simulink model "MicrogridControl"  (R2025b)
settings: Solver=VariableStepAuto  StartTime=0.0  StopTime=8  FixedStep=Ts  RelTol=1e-3
PreLoadFcn:
  | NormalOperation;
  | MicrogridControlParam;
undefined symbols (not defined in the file): base, bessModeInitial, bessSystem, bessVoltage, breakerStatus, DiscIntNeverNeededParam, ee_sli_rtmsupport, event, gcbh, generator, gflInverter, gfmInverter, Inertia, lineInductance, lineResistance, machine, plannedIsland, pmsm, powerLimit, powerQuality, PV, PVInverter, ref, resync, solar, solarInsolationChange, systemFrequency, Ts, windController, windSystem, windTurbine
libraries: nesl_utility x234, ee_lib x174, fl_lib x143, eeGeneralControl x137, simulink x78, eeTransforms x47, slpidlib x23, nesl_utility_internal x12, eePwmGenerator x9, eeSinusoidalMeasurementV2 x9, custom_lib x7, batteryecm_lib x6
(part 1 of 25)
settings Model: SimulationMode=accelerator  Creator=skota  LastModifiedBy=skota
settings DataIOCC: SaveOutput=off  DSMLogging=off  SaveTime=off  ReturnWorkspaceOutputs=off
settings DebuggingCC: MinStepSizeMsg=none  FrameProcessingCompatibilityMsg=none
settings SimscapeCC: SimscapeNormalizeSystem=off

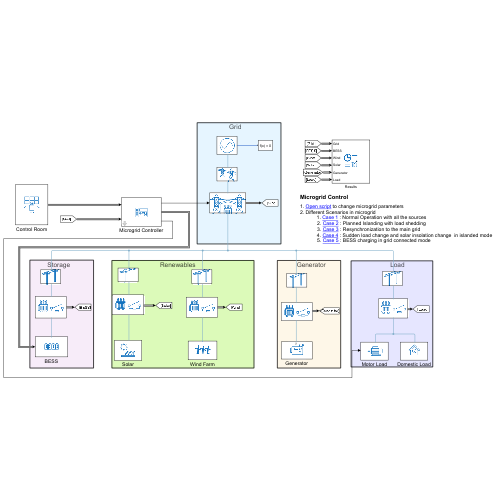
[thumbnail: Simulink's stored preview of the top-level diagram]
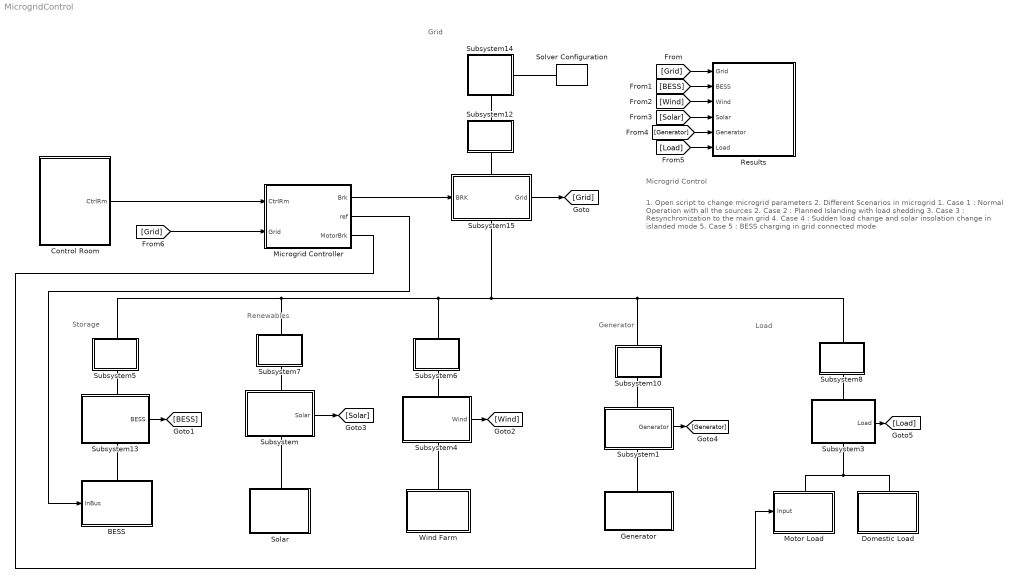
== system MicrogridControl ==
  note: Renewables
  note: Storage
  note: Generator
  note: Load
  note: Grid
  note: 1. Open script to change microgrid parameters
      | 2. Different Scenarios in microgrid
      | 1. Case 1 : Normal Operation with all the sources
      | 2. Case 2 : Planned Islanding with load shedding
      | 3. Case 3 : Resynchronization to the main grid
      | 4. Case 4 : Sudden load change and solar insolation change in islanded mode
      | 5. Case 5 : BESS charging in grid connected mode
  note: Microgrid Control
  BESS : Subsystem
      settings: PortSchema="{\"entries\":[{\"content\":{\"sides\":[{\"content\":{\"connectorIds\":[\"In1\"]},\"type\":\"ConnectorPlacement.EquallySpacedRectSide\",\"uuid\":\"138c02f1-8438-4b9e-be08-ceaf3940f6c7\"},{\"content\":{\"side\":\"RIGHT\"},\"type\":\"ConnectorPlacement.EquallySpacedRectSide\",\"uuid\":\"34af79ec-6d74-4c96-bf33-cc8e5a370ddd\"},{\"content\":{\"connectorIds\":[\"LConn1\"],\"side\":\"TOP\"},\"type\":\"ConnectorPlacement.EquallySpacedRectSide\",\"uuid\":\"48313b6e-1835-49d8-b154-057b5fb517b0\"}]},\"type\":\"ConnectorPlacement.EquallySpacedConnector\",\"uuid\":\"b091f0a3-fffe-4dfb-8622-14774ce4c9e9\"}],\"packageUris\":[\"http://schema.mathworks.com/mf0/Connector/R2020b\"],\"version\":\"1.0\"}"
  Control Room : Subsystem
  Domestic Load : Subsystem
      settings: PortSchema="{\"entries\":[{\"content\":{\"sides\":[{\"content\":{},\"type\":\"ConnectorPlacement.EquallySpacedRectSide\",\"uuid\":\"f8fc4132-7548-4a0f-8659-b0fbdf7b43f6\"},{\"content\":{\"side\":\"RIGHT\"},\"type\":\"ConnectorPlacement.EquallySpacedRectSide\",\"uuid\":\"c12bc99a-3747-4ef2-b83e-90fecef76ea5\"},{\"content\":{\"connectorIds\":[\"LConn1\"],\"side\":\"TOP\"},\"type\":\"ConnectorPlacement.EquallySpacedRectSide\",\"uuid\":\"28127f01-067a-40fd-84ae-a789b4333a80\"}]},\"type\":\"ConnectorPlacement.EquallySpacedConnector\",\"uuid\":\"c6f5d860-c088-4c19-8c9a-849451abfa64\"}],\"packageUris\":[\"http://schema.mathworks.com/mf0/Connector/R2020b\"],\"version\":\"1.0\"}"
  Generator : Subsystem
      settings: PortSchema="{\"entries\":[{\"content\":{\"sides\":[{\"content\":{},\"type\":\"ConnectorPlacement.EquallySpacedRectSide\",\"uuid\":\"0e4bb094-5f01-4715-b678-e6b326bbface\"},{\"content\":{\"side\":\"RIGHT\"},\"type\":\"ConnectorPlacement.EquallySpacedRectSide\",\"uuid\":\"0cb60177-20db-48f9-a9cc-070daf12251a\"},{\"content\":{\"connectorIds\":[\"LConn1\"],\"side\":\"TOP\"},\"type\":\"ConnectorPlacement.EquallySpacedRectSide\",\"uuid\":\"205cef4a-01a9-469e-ade5-58cd4fb704d4\"},{\"content\":{\"side\":\"BOTTOM\"},\"type\":\"ConnectorPlacement.EquallySpacedRectSide\",\"uuid\":\"006e0ade-b558-4494-a2f0-eb5d5c15551c\"}]},\"type\":\"ConnectorPlacement.EquallySpacedConnector\",\"uuid\":\"9a4799c2-8742-4ae9-b78d-c2acced826f3\"}],\"packageUris\":[\"http://schema.mathworks.com/mf0/Connector/R2020b\"],\"version\":\"1.0\"}"
  Microgrid Controller : Subsystem  mask{resynchronization=on, plannedIslanding=on, blackStart=on, kpPLL=40, kiPLL=1000, frequencyPLL=systemFrequency, sampleTimePLL=Ts, pUpperLimit=powerLimit.upper, pLowerLimit=powerLimit.lower, qUpperLimit=powerLimit.upper, qLowerLimit=powerLimit.lower, gridFrequency=systemFrequency, resyncDelay=resync.delay, kpVoltage=resync.kpVoltage, kiVoltage=resync.kiVoltage, voltageThreshold=resync.vThreshold, voltageDroop=resync.vDroop, kpFrequency=resync.kpFrequency, kiFrequency=resync.kiFrequency, frequencyThreshold=resync.fThreshold, kpAngle=resync.kpAngle, kiAngle=resync.kiAngle, angleThreshold=resync.aThreshold, plannedIslandingDelay=plannedIsland.delay, kpActive=plannedIsland.kPActive, kiActive=plannedIsland.kIActive, activeThreshold=plannedIsland.pThreshold, kpReactive=plannedIsland.kPReactive, kiReactive=plannedIsland.kiReactive, reactiveThreshold=plannedIsland.qThreshold, blackStartTime=1000, blackStartFrequency=50, level1=0.1, level2=0.2, level3=0.7, delay1=1, delay2=2, delay3=3, upperVoltagelimit=powerQuality.maxVoltage, lowerVoltageLimit=powerQuality.minVoltage, upperFrequencyLimit=powerQuality.maxFrequency, lowerFrequencyLimit=powerQuality.minFrequency}
      mask prompts: plannedIslanding "Planned Islanding"; blackStart "Black Start"; kpPLL "Proportional Gain"; kiPLL "Integral Gain"; frequencyPLL "Grid Frequency in Hz"; sampleTimePLL "Sample Time in sec"; pUpperLimit "Upper Limit in pu"; pLowerLimit "Lower Limit in pu"; qUpperLimit "Upper Limit in pu"; qLowerLimit "Lower Limit in pu"; gridFrequency "Grid Frequency in Hz"; resyncDelay "Resynchronization delay in sec"; kpVoltage "Proportional Gain"; kiVoltage "Voltage Integral Gain"; voltageThreshold "Threshold"; voltageDroop "Reactive Power Droop"; kpFrequency "Proportional Gain"; kiFrequency "Integral Gain"; frequencyThreshold "Threshold"; kpAngle "Proportional Gain"; kiAngle "Integral Gain"; angleThreshold "Threshold"; plannedIslandingDelay "Delay in sec"; kpActive "Proportional Gain"; kiActive "Integral Gain"; activeThreshold "Threshold"; kpReactive "Proportional Gain"; kiReactive "Integral Gain"; reactiveThreshold "Threshold"; blackStartTime "Black Start Time in sec"; blackStartFrequency "Reference Frequency in Hz"; level1 "Level 1 in pu"; level2 "Level 2 in pu"; level3 "Level 3 in pu"; delay1 "Delay 1 in sec"; delay2 "Delay2 in sec"; delay3 "Delay3 in sec"; upperVoltagelimit "Maximum Voltage in pu"; lowerVoltageLimit "Minimum Voltage in pu"; upperFrequencyLimit "Maximum frequency in Hz"; lowerFrequencyLimit "Minimum Frequency in Hz"
      mask init:
      | plannedIslandingBlock = [gcb,'/','Microgrid Control Functions','/','Planned Islanding'];
      | resynchBlock = [gcb,'/','Microgrid Control Functions','/','Resynchronization'];
      | blackStartBlock = [gcb,'/','Microgrid Control Functions','/','Black Start'];
      | block = {resynchBlock,plannedIslandingBlock,blackStartBlock};
      | blockEnable = {get_param(gcb,'resynchronization'),get_param(gcb,'plannedIslanding'),get_param(gcb,'blackStart')};
      | parameterIdx = {12:23,24:30,31:38};
      | % Set the 'MaskVisibilities' property for each parameters
      | cArray=cell(1,42);
      | cArray(:)={'on'};
      | for blockIdx = 1:length(block)
      |     if strcmp(blockEnable{blockIdx},'on')
      |         cArray(parameterIdx{blockIdx}) = {'on'};
      |     else
      |         cArray(parameterIdx{blockIdx}) = {'off'};
      |     end
      | end
      | set_param(gcb,'MaskVisibilities',cArray);
      mask Callback resynchronization:
      | plannedIslandingBlock = [gcb,'/','Microgrid Control Functions','/','Planned Islanding'];
      | resynchBlock = [gcb,'/','Microgrid Control Functions','/','Resynchronization'];
      | blackStartBlock = [gcb,'/','Microgrid Control Functions','/','Black Start'];
      | block = {resynchBlock,plannedIslandingBlock,blackStartBlock};
      | blockEnable = {get_param(gcb,'resynchronization'),get_param(gcb,'plannedIslanding'),get_param(gcb,'blackStart')};
      | parameterIdx = {12:23,24:30,31:38};
      | % Set the 'MaskVisibilities' property for each parameters
      | cArray=cell(1,42);
      | cArray(:)={'on'};
      | for blockIdx = 1:length(block)
      |     if strcmp(blockEnable{blockIdx},'on')
      |         cArray(parameterIdx{blockIdx}) = {'on'};
      |     else
      |         cArray(parameterIdx{blockIdx}) = {'off'};
      |     end
      | end
      | set_param(gcb,'MaskVisibilities',cArray);
      mask Callback plannedIslanding:
      | plannedIslandingBlock = [gcb,'/','Microgrid Control Functions','/','Planned Islanding'];
      | resynchBlock = [gcb,'/','Microgrid Control Functions','/','Resynchronization'];
      | blackStartBlock = [gcb,'/','Microgrid Control Functions','/','Black Start'];
      | block = {resynchBlock,plannedIslandingBlock,blackStartBlock};
      | blockEnable = {get_param(gcb,'resynchronization'),get_param(gcb,'plannedIslanding'),get_param(gcb,'blackStart')};
      | parameterIdx = {12:23,24:30,31:38};
      | % Set the 'MaskVisibilities' property for each parameters
      | cArray=cell(1,42);
      | cArray(:)={'on'};
      | for blockIdx = 1:length(block)
      |     if strcmp(blockEnable{blockIdx},'on')
      |         cArray(parameterIdx{blockIdx}) = {'on'};
      |     else
      |         cArray(parameterIdx{blockIdx}) = {'off'};
      |     end
      | end
      | set_param(gcb,'MaskVisibilities',cArray);
      mask Callback blackStart:
      | plannedIslandingBlock = [gcb,'/','Microgrid Control Functions','/','Planned Islanding'];
      | resynchBlock = [gcb,'/','Microgrid Control Functions','/','Resynchronization'];
      | blackStartBlock = [gcb,'/','Microgrid Control Functions','/','Black Start'];
      | block = {resynchBlock,plannedIslandingBlock,blackStartBlock};
      | blockEnable = {get_param(gcb,'resynchronization'),get_param(gcb,'plannedIslanding'),get_param(gcb,'blackStart')};
      | parameterIdx = {12:23,24:30,31:38};
      | % Set the 'MaskVisibilities' property for each parameters
      | cArray=cell(1,42);
      | cArray(:)={'on'};
      | for blockIdx = 1:length(block)
      |     if strcmp(blockEnable{blockIdx},'on')
      |         cArray(parameterIdx{blockIdx}) = {'on'};
      |     else
      |         cArray(parameterIdx{blockIdx}) = {'off'};
      |     end
      | end
      | set_param(gcb,'MaskVisibilities',cArray);
      mask DialogControl ParameterGroupVar Prompt: Microgrid control functions
      mask DialogControl Container22 Prompt: PLL
      mask DialogControl Container25 Prompt: General
      mask DialogControl Container23 Prompt: Reference Generation
      mask DialogControl Container27 Prompt: Active Power
      mask DialogControl Container28 Prompt: Reactive Power
      mask DialogControl Container3 Prompt: Resynchronization
      mask DialogControl Container15 Prompt: General
      mask DialogControl Container9 Prompt: Voltage
      mask DialogControl Container10 Prompt: Frequency
      mask DialogControl Container11 Prompt: Angle
      mask DialogControl Container8 Prompt: Planned Islanding
      mask DialogControl Container16 Prompt: General
      mask DialogControl Container13 Prompt: Active Power
      mask DialogControl Container14 Prompt: Reactive Power
      mask DialogControl Container17 Prompt: Black Start
      mask DialogControl Container19 Prompt: General
      mask DialogControl Container20 Prompt: Voltage Levels
      mask DialogControl Container21 Prompt: Time Delays
      mask DialogControl Container261 Prompt: Power Quality Metrics
  Motor Load : Subsystem
      settings: PortSchema="{\"entries\":[{\"content\":{\"sides\":[{\"content\":{\"connectorIds\":[\"In1\"]},\"type\":\"ConnectorPlacement.EquallySpacedRectSide\",\"uuid\":\"f8fc4132-7548-4a0f-8659-b0fbdf7b43f6\"},{\"content\":{\"side\":\"RIGHT\"},\"type\":\"ConnectorPlacement.EquallySpacedRectSide\",\"uuid\":\"c12bc99a-3747-4ef2-b83e-90fecef76ea5\"},{\"content\":{\"connectorIds\":[\"LConn1\"],\"side\":\"TOP\"},\"type\":\"ConnectorPlacement.EquallySpacedRectSide\",\"uuid\":\"28127f01-067a-40fd-84ae-a789b4333a80\"}]},\"type\":\"ConnectorPlacement.EquallySpacedConnector\",\"uuid\":\"c6f5d860-c088-4c19-8c9a-849451abfa64\"}],\"packageUris\":[\"http://schema.mathworks.com/mf0/Connector/R2020b\"],\"version\":\"1.0\"}"
  Results : Subsystem
  Solar : Subsystem
      settings: PortSchema="{\"entries\":[{\"content\":{\"sides\":[{\"content\":{},\"type\":\"ConnectorPlacement.EquallySpacedRectSide\",\"uuid\":\"138c02f1-8438-4b9e-be08-ceaf3940f6c7\"},{\"content\":{\"side\":\"RIGHT\"},\"type\":\"ConnectorPlacement.EquallySpacedRectSide\",\"uuid\":\"34af79ec-6d74-4c96-bf33-cc8e5a370ddd\"},{\"content\":{\"connectorIds\":[\"LConn1\"],\"side\":\"TOP\"},\"type\":\"ConnectorPlacement.EquallySpacedRectSide\",\"uuid\":\"48313b6e-1835-49d8-b154-057b5fb517b0\"}]},\"type\":\"ConnectorPlacement.EquallySpacedConnector\",\"uuid\":\"b091f0a3-fffe-4dfb-8622-14774ce4c9e9\"}],\"packageUris\":[\"http://schema.mathworks.com/mf0/Connector/R2020b\"],\"version\":\"1.0\"}"
  Solver Configuration : nesl_utility/Solver Configuration  PhysicalDomain=network_engine_domain  SubClassName=solver  LeftPortType=input  RightPortType=generic  Tones=[]  Harmonics=[]  SimulateNoise=off  Profile=off  UseLocalSampling=off  EnableSwitchedLinearOptims=on  FrequencyDomain=off  UseCCode=off  RelTol=0.001  AbsTol=0.001  MinStep=1e-09  ToWorkspace=off  RevertToSquareIcSolve=off  NumHomotopyIterations=100  PhasorMode=off  PhasorModeNumHarmonics=1  ConsistencySolver=NEWTON_XTOL_AFTER_FTOL  IndexReductionMethod=None  DoDC=off  ResidualTolerance=1e-09  ConsistencyTolSource=GLOBAL  ConsistencyAbsTol=0.001  ConsistencyRelTol=0.001  ConsistencyTolFactor=1e3  UseLocalSolver=on  LocalSolverChoice=NE_BACKWARD_EULER_ADVANCER  ResolveIndetEquations=off  FunctionEvalNumThread=1  LocalSolverSampleTime=5e-05  DoFixedCost=on  MaxNonlinIter=1  MaxModeIter=2  ComputeImpulses=off  ImpulseIterations=2  LinearAlgebra=Sparse  LinearAlgebraNumThread=0  EquationFormulation=NE_TIME_EF  DelaysMemoryBudget=1024  AutomaticFiltering=off  FilteringTimeConstant=0.001  PartitionStorageMethod=AS_NEEDED  PartitionMemoryBudget=1024  PartitionMethod=ROBUST  MultibodyUseLocalSolver=off  MultibodyLocalSolverChoice=ODE1  MultibodyLocalSolverSampleTime=0.001
  Subsystem : Subsystem
      settings: PortSchema="{\"entries\":[{\"content\":{\"sides\":[{\"content\":{},\"type\":\"ConnectorPlacement.EquallySpacedRectSide\",\"uuid\":\"075ebd5a-6b04-48de-85cd-c24816f3ab65\"},{\"content\":{\"connectorIds\":[\"Out1\"],\"side\":\"RIGHT\"},\"type\":\"ConnectorPlacement.EquallySpacedRectSide\",\"uuid\":\"41ac91c2-3615-4598-a46d-cbf5e56a9c7c\"},{\"content\":{\"connectorIds\":[\"LConn1\"],\"side\":\"TOP\"},\"type\":\"ConnectorPlacement.EquallySpacedRectSide\",\"uuid\":\"e69c000e-49b0-47b4-a3d7-4acaa4ad1562\"},{\"content\":{\"connectorIds\":[\"RConn1\"],\"side\":\"BOTTOM\"},\"type\":\"ConnectorPlacement.EquallySpacedRectSide\",\"uuid\":\"b492b74c-ffe9-47f0-b730-c4df118b748d\"}]},\"type\":\"ConnectorPlacement.EquallySpacedConnector\",\"uuid\":\"0905c5bd-be34-4bdd-a956-be8a26354884\"}],\"packageUris\":[\"http://schema.mathworks.com/mf0/Connector/R2020b\"],\"version\":\"1.0\"}"
  Subsystem1 : Subsystem
      settings: PortSchema="{\"entries\":[{\"content\":{\"sides\":[{\"content\":{},\"type\":\"ConnectorPlacement.EquallySpacedRectSide\",\"uuid\":\"075ebd5a-6b04-48de-85cd-c24816f3ab65\"},{\"content\":{\"connectorIds\":[\"Out1\"],\"side\":\"RIGHT\"},\"type\":\"ConnectorPlacement.EquallySpacedRectSide\",\"uuid\":\"41ac91c2-3615-4598-a46d-cbf5e56a9c7c\"},{\"content\":{\"connectorIds\":[\"LConn1\"],\"side\":\"TOP\"},\"type\":\"ConnectorPlacement.EquallySpacedRectSide\",\"uuid\":\"e69c000e-49b0-47b4-a3d7-4acaa4ad1562\"},{\"content\":{\"connectorIds\":[\"RConn1\"],\"side\":\"BOTTOM\"},\"type\":\"ConnectorPlacement.EquallySpacedRectSide\",\"uuid\":\"96b4f92e-fe79-4635-adc4-53c284aabfb3\"}]},\"type\":\"ConnectorPlacement.EquallySpacedConnector\",\"uuid\":\"0905c5bd-be34-4bdd-a956-be8a26354884\"}],\"packageUris\":[\"http://schema.mathworks.com/mf0/Connector/R2020b\"],\"version\":\"1.0\"}"
  Subsystem10 : Subsystem
      settings: PortSchema="{\"entries\":[{\"content\":{\"sides\":[{\"content\":{},\"type\":\"ConnectorPlacement.EquallySpacedRectSide\",\"uuid\":\"b9f8da2b-6ad0-442d-bcb1-cc8d78629a21\"},{\"content\":{\"side\":\"RIGHT\"},\"type\":\"ConnectorPlacement.EquallySpacedRectSide\",\"uuid\":\"5098ade6-5e08-47f7-aaf7-f83895131c9a\"},{\"content\":{\"connectorIds\":[\"LConn1\"],\"side\":\"TOP\"},\"type\":\"ConnectorPlacement.EquallySpacedRectSide\",\"uuid\":\"1f29bdb1-48b4-4502-a518-a8a9b6cf9387\"},{\"content\":{\"connectorIds\":[\"RConn1\"],\"side\":\"BOTTOM\"},\"type\":\"ConnectorPlacement.EquallySpacedRectSide\",\"uuid\":\"2fa4a532-6b46-462a-9006-dc12ce35ad72\"}]},\"type\":\"ConnectorPlacement.EquallySpacedConnector\",\"uuid\":\"eec1a01f-afa1-4be0-9c9d-9922ab640285\"}],\"packageUris\":[\"http://schema.mathworks.com/mf0/Connector/R2020b\"],\"version\":\"1.0\"}"
  Subsystem12 : Subsystem
      settings: PortSchema="{\"entries\":[{\"content\":{\"sides\":[{\"content\":{},\"type\":\"ConnectorPlacement.EquallySpacedRectSide\",\"uuid\":\"b9f8da2b-6ad0-442d-bcb1-cc8d78629a21\"},{\"content\":{\"side\":\"RIGHT\"},\"type\":\"ConnectorPlacement.EquallySpacedRectSide\",\"uuid\":\"5098ade6-5e08-47f7-aaf7-f83895131c9a\"},{\"content\":{\"connectorIds\":[\"LConn1\"],\"side\":\"TOP\"},\"type\":\"ConnectorPlacement.EquallySpacedRectSide\",\"uuid\":\"1f29bdb1-48b4-4502-a518-a8a9b6cf9387\"},{\"content\":{\"connectorIds\":[\"RConn1\"],\"side\":\"BOTTOM\"},\"type\":\"ConnectorPlacement.EquallySpacedRectSide\",\"uuid\":\"c3a9824f-a87f-472d-814a-dea79d7ebb6e\"}]},\"type\":\"ConnectorPlacement.EquallySpacedConnector\",\"uuid\":\"eec1a01f-afa1-4be0-9c9d-9922ab640285\"}],\"packageUris\":[\"http://schema.mathworks.com/mf0/Connector/R2020b\"],\"version\":\"1.0\"}"
  Subsystem13 : Subsystem
      settings: PortSchema="{\"entries\":[{\"content\":{\"sides\":[{\"content\":{},\"type\":\"ConnectorPlacement.EquallySpacedRectSide\",\"uuid\":\"075ebd5a-6b04-48de-85cd-c24816f3ab65\"},{\"content\":{\"connectorIds\":[\"Out1\"],\"side\":\"RIGHT\"},\"type\":\"ConnectorPlacement.EquallySpacedRectSide\",\"uuid\":\"41ac91c2-3615-4598-a46d-cbf5e56a9c7c\"},{\"content\":{\"connectorIds\":[\"LConn1\"],\"side\":\"TOP\"},\"type\":\"ConnectorPlacement.EquallySpacedRectSide\",\"uuid\":\"e69c000e-49b0-47b4-a3d7-4acaa4ad1562\"},{\"content\":{\"connectorIds\":[\"RConn1\"],\"side\":\"BOTTOM\"},\"type\":\"ConnectorPlacement.EquallySpacedRectSide\",\"uuid\":\"77ad34f3-1b61-4e3d-a649-9106eae34ef8\"}]},\"type\":\"ConnectorPlacement.EquallySpacedConnector\",\"uuid\":\"0905c5bd-be34-4bdd-a956-be8a26354884\"}],\"packageUris\":[\"http://schema.mathworks.com/mf0/Connector/R2020b\"],\"version\":\"1.0\"}"
  Subsystem14 : Subsystem
      settings: PortSchema="{\"entries\":[{\"content\":{\"sides\":[{\"content\":{\"connectorIds\":[\"LConn1\"]},\"type\":\"ConnectorPlacement.EquallySpacedRectSide\",\"uuid\":\"b9f8da2b-6ad0-442d-bcb1-cc8d78629a21\"},{\"content\":{\"side\":\"RIGHT\"},\"type\":\"ConnectorPlacement.EquallySpacedRectSide\",\"uuid\":\"5098ade6-5e08-47f7-aaf7-f83895131c9a\"},{\"content\":{\"side\":\"TOP\"},\"type\":\"ConnectorPlacement.EquallySpacedRectSide\",\"uuid\":\"1f29bdb1-48b4-4502-a518-a8a9b6cf9387\"},{\"content\":{\"connectorIds\":[\"RConn1\"],\"side\":\"BOTTOM\"},\"type\":\"ConnectorPlacement.EquallySpacedRectSide\",\"uuid\":\"873d74d6-765d-4285-8db4-ddaebfd01f7f\"}]},\"type\":\"ConnectorPlacement.EquallySpacedConnector\",\"uuid\":\"eec1a01f-afa1-4be0-9c9d-9922ab640285\"}],\"packageUris\":[\"http://schema.mathworks.com/mf0/Connector/R2020b\"],\"version\":\"1.0\"}"
  Subsystem15 : Subsystem
      settings: PortSchema="{\"entries\":[{\"content\":{\"sides\":[{\"content\":{\"connectorIds\":[\"In1\"]},\"type\":\"ConnectorPlacement.EquallySpacedRectSide\",\"uuid\":\"075ebd5a-6b04-48de-85cd-c24816f3ab65\"},{\"content\":{\"connectorIds\":[\"Out1\"],\"side\":\"RIGHT\"},\"type\":\"ConnectorPlacement.EquallySpacedRectSide\",\"uuid\":\"41ac91c2-3615-4598-a46d-cbf5e56a9c7c\"},{\"content\":{\"connectorIds\":[\"LConn1\"],\"side\":\"TOP\"},\"type\":\"ConnectorPlacement.EquallySpacedRectSide\",\"uuid\":\"e69c000e-49b0-47b4-a3d7-4acaa4ad1562\"},{\"content\":{\"connectorIds\":[\"RConn1\"],\"side\":\"BOTTOM\"},\"type\":\"ConnectorPlacement.EquallySpacedRectSide\",\"uuid\":\"7ae2fdc1-c7d6-46e9-8430-7e355503bf0c\"}]},\"type\":\"ConnectorPlacement.EquallySpacedConnector\",\"uuid\":\"0905c5bd-be34-4bdd-a956-be8a26354884\"}],\"packageUris\":[\"http://schema.mathworks.com/mf0/Connector/R2020b\"],\"version\":\"1.0\"}"
  Subsystem3 : Subsystem
      settings: PortSchema="{\"entries\":[{\"content\":{\"sides\":[{\"content\":{},\"type\":\"ConnectorPlacement.EquallySpacedRectSide\",\"uuid\":\"075ebd5a-6b04-48de-85cd-c24816f3ab65\"},{\"content\":{\"connectorIds\":[\"Out1\"],\"side\":\"RIGHT\"},\"type\":\"ConnectorPlacement.EquallySpacedRectSide\",\"uuid\":\"41ac91c2-3615-4598-a46d-cbf5e56a9c7c\"},{\"content\":{\"connectorIds\":[\"LConn1\"],\"side\":\"TOP\"},\"type\":\"ConnectorPlacement.EquallySpacedRectSide\",\"uuid\":\"e69c000e-49b0-47b4-a3d7-4acaa4ad1562\"},{\"content\":{\"connectorIds\":[\"RConn1\"],\"side\":\"BOTTOM\"},\"type\":\"ConnectorPlacement.EquallySpacedRectSide\",\"uuid\":\"a7c18ddf-0715-43ed-9a8b-b9971972e837\"}]},\"type\":\"ConnectorPlacement.EquallySpacedConnector\",\"uuid\":\"0905c5bd-be34-4bdd-a956-be8a26354884\"}],\"packageUris\":[\"http://schema.mathworks.com/mf0/Connector/R2020b\"],\"version\":\"1.0\"}"
  Subsystem4 : Subsystem
      settings: PortSchema="{\"entries\":[{\"content\":{\"sides\":[{\"content\":{},\"type\":\"ConnectorPlacement.EquallySpacedRectSide\",\"uuid\":\"075ebd5a-6b04-48de-85cd-c24816f3ab65\"},{\"content\":{\"connectorIds\":[\"Out1\"],\"side\":\"RIGHT\"},\"type\":\"ConnectorPlacement.EquallySpacedRectSide\",\"uuid\":\"41ac91c2-3615-4598-a46d-cbf5e56a9c7c\"},{\"content\":{\"connectorIds\":[\"LConn1\"],\"side\":\"TOP\"},\"type\":\"ConnectorPlacement.EquallySpacedRectSide\",\"uuid\":\"e69c000e-49b0-47b4-a3d7-4acaa4ad1562\"},{\"content\":{\"connectorIds\":[\"RConn1\"],\"side\":\"BOTTOM\"},\"type\":\"ConnectorPlacement.EquallySpacedRectSide\",\"uuid\":\"4a1785f3-ca3e-404d-af4e-553346c14799\"}]},\"type\":\"ConnectorPlacement.EquallySpacedConnector\",\"uuid\":\"0905c5bd-be34-4bdd-a956-be8a26354884\"}],\"packageUris\":[\"http://schema.mathworks.com/mf0/Connector/R2020b\"],\"version\":\"1.0\"}"
  Subsystem5 : Subsystem
      settings: PortSchema="{\"entries\":[{\"content\":{\"sides\":[{\"content\":{},\"type\":\"ConnectorPlacement.EquallySpacedRectSide\",\"uuid\":\"b9f8da2b-6ad0-442d-bcb1-cc8d78629a21\"},{\"content\":{\"side\":\"RIGHT\"},\"type\":\"ConnectorPlacement.EquallySpacedRectSide\",\"uuid\":\"5098ade6-5e08-47f7-aaf7-f83895131c9a\"},{\"content\":{\"connectorIds\":[\"LConn1\"],\"side\":\"TOP\"},\"type\":\"ConnectorPlacement.EquallySpacedRectSide\",\"uuid\":\"1f29bdb1-48b4-4502-a518-a8a9b6cf9387\"},{\"content\":{\"connectorIds\":[\"RConn1\"],\"side\":\"BOTTOM\"},\"type\":\"ConnectorPlacement.EquallySpacedRectSide\",\"uuid\":\"cfc0c68d-8b97-48cb-b358-ec38e6134a86\"}]},\"type\":\"ConnectorPlacement.EquallySpacedConnector\",\"uuid\":\"eec1a01f-afa1-4be0-9c9d-9922ab640285\"}],\"packageUris\":[\"http://schema.mathworks.com/mf0/Connector/R2020b\"],\"version\":\"1.0\"}"
  Subsystem6 : Subsystem
      settings: PortSchema="{\"entries\":[{\"content\":{\"sides\":[{\"content\":{},\"type\":\"ConnectorPlacement.EquallySpacedRectSide\",\"uuid\":\"b9f8da2b-6ad0-442d-bcb1-cc8d78629a21\"},{\"content\":{\"side\":\"RIGHT\"},\"type\":\"ConnectorPlacement.EquallySpacedRectSide\",\"uuid\":\"5098ade6-5e08-47f7-aaf7-f83895131c9a\"},{\"content\":{\"connectorIds\":[\"LConn1\"],\"side\":\"TOP\"},\"type\":\"ConnectorPlacement.EquallySpacedRectSide\",\"uuid\":\"1f29bdb1-48b4-4502-a518-a8a9b6cf9387\"},{\"content\":{\"connectorIds\":[\"RConn1\"],\"side\":\"BOTTOM\"},\"type\":\"ConnectorPlacement.EquallySpacedRectSide\",\"uuid\":\"2f9dfb11-72c9-4c7c-b594-dea004a9b391\"}]},\"type\":\"ConnectorPlacement.EquallySpacedConnector\",\"uuid\":\"eec1a01f-afa1-4be0-9c9d-9922ab640285\"}],\"packageUris\":[\"http://schema.mathworks.com/mf0/Connector/R2020b\"],\"version\":\"1.0\"}"
  Subsystem7 : Subsystem
      settings: PortSchema="{\"entries\":[{\"content\":{\"sides\":[{\"content\":{},\"type\":\"ConnectorPlacement.EquallySpacedRectSide\",\"uuid\":\"b9f8da2b-6ad0-442d-bcb1-cc8d78629a21\"},{\"content\":{\"side\":\"RIGHT\"},\"type\":\"ConnectorPlacement.EquallySpacedRectSide\",\"uuid\":\"5098ade6-5e08-47f7-aaf7-f83895131c9a\"},{\"content\":{\"connectorIds\":[\"LConn1\"],\"side\":\"TOP\"},\"type\":\"ConnectorPlacement.EquallySpacedRectSide\",\"uuid\":\"1f29bdb1-48b4-4502-a518-a8a9b6cf9387\"},{\"content\":{\"connectorIds\":[\"RConn1\"],\"side\":\"BOTTOM\"},\"type\":\"ConnectorPlacement.EquallySpacedRectSide\",\"uuid\":\"e81e4011-f04d-4084-ada3-8cdb0095883a\"}]},\"type\":\"ConnectorPlacement.EquallySpacedConnector\",\"uuid\":\"eec1a01f-afa1-4be0-9c9d-9922ab640285\"}],\"packageUris\":[\"http://schema.mathworks.com/mf0/Connector/R2020b\"],\"version\":\"1.0\"}"
  Subsystem8 : Subsystem
      settings: PortSchema="{\"entries\":[{\"content\":{\"sides\":[{\"content\":{},\"type\":\"ConnectorPlacement.EquallySpacedRectSide\",\"uuid\":\"b9f8da2b-6ad0-442d-bcb1-cc8d78629a21\"},{\"content\":{\"side\":\"RIGHT\"},\"type\":\"ConnectorPlacement.EquallySpacedRectSide\",\"uuid\":\"5098ade6-5e08-47f7-aaf7-f83895131c9a\"},{\"content\":{\"connectorIds\":[\"LConn1\"],\"side\":\"TOP\"},\"type\":\"ConnectorPlacement.EquallySpacedRectSide\",\"uuid\":\"1f29bdb1-48b4-4502-a518-a8a9b6cf9387\"},{\"content\":{\"connectorIds\":[\"RConn1\"],\"side\":\"BOTTOM\"},\"type\":\"ConnectorPlacement.EquallySpacedRectSide\",\"uuid\":\"d9e19b97-7210-4386-8816-c47a633945c3\"}]},\"type\":\"ConnectorPlacement.EquallySpacedConnector\",\"uuid\":\"eec1a01f-afa1-4be0-9c9d-9922ab640285\"}],\"packageUris\":[\"http://schema.mathworks.com/mf0/Connector/R2020b\"],\"version\":\"1.0\"}"
  Wind Farm : Subsystem
      settings: PortSchema="{\"entries\":[{\"content\":{\"sides\":[{\"content\":{},\"type\":\"ConnectorPlacement.EquallySpacedRectSide\",\"uuid\":\"d3659d2d-402c-4ee1-9775-2e102b20ba17\"},{\"content\":{\"side\":\"RIGHT\"},\"type\":\"ConnectorPlacement.EquallySpacedRectSide\",\"uuid\":\"af063bca-5841-4f29-980e-f2cabf147052\"},{\"content\":{\"connectorIds\":[\"LConn1\"],\"side\":\"TOP\"},\"type\":\"ConnectorPlacement.EquallySpacedRectSide\",\"uuid\":\"07dd149e-b476-4027-b937-3b1b12a367ee\"}]},\"type\":\"ConnectorPlacement.EquallySpacedConnector\",\"uuid\":\"d2793dbd-467d-413f-837e-73430b2f2381\"}],\"packageUris\":[\"http://schema.mathworks.com/mf0/Connector/R2020b\"],\"version\":\"1.0\"}"
  wires:
  [BESS] -> Results/2(BESS)
  Microgrid Controller/1(Brk) -> Subsystem15/1(BRK)
  Subsystem15/1(Grid) -> [Grid]
  Subsystem3/1(Load) -> [Load]
  Microgrid Controller/3(MotorBrk) -> Motor Load/1(Input)
  [Wind] -> Results/3(Wind)
  [Grid] -> Microgrid Controller/2(Grid)
  Subsystem/1(Solar) -> [Solar]
  Control Room/1(CtrlRm) -> Microgrid Controller/1(CtrlRm)
  Subsystem1/1(Generator) -> [Generator]
  [Generator] -> Results/5(Generator)
  [Solar] -> Results/4(Solar)
  Subsystem13/1(BESS) -> [BESS]
  [Load] -> Results/6(Load)
  Subsystem4/1(Wind) -> [Wind]
  [Grid] -> Results/1(Grid)
  Microgrid Controller/2(ref) -> BESS/1(InBus)
  connections:
  Subsystem7/LConn1 -- Subsystem15/RConn1 -- Subsystem8/LConn1 -- Subsystem10/LConn1 -- Subsystem6/LConn1 -- Subsystem5/LConn1
  Domestic Load/LConn1 -- Motor Load/LConn1 -- Subsystem3/RConn1
  Subsystem14/LConn1 -- Solver Configuration/RConn1
  Subsystem10/RConn1 -- Subsystem1/LConn1
  Subsystem6/RConn1 -- Subsystem4/LConn1
  Subsystem5/RConn1 -- Subsystem13/LConn1
  Generator/LConn1 -- Subsystem1/RConn1
  Subsystem15/LConn1 -- Subsystem12/RConn1
  Subsystem8/RConn1 -- Subsystem3/LConn1
  Subsystem14/RConn1 -- Subsystem12/LConn1
  Wind Farm/LConn1 -- Subsystem4/RConn1
  Subsystem7/RConn1 -- Subsystem/LConn1
  Subsystem/RConn1 -- Solar/LConn1
  Subsystem13/RConn1 -- BESS/LConn1
